simulink model "AircraftModel_LonMot"  (R2020b)
settings: Solver=VariableStepAuto  StartTime=0.0  StopTime=2000  FixedStep=CNT_StepSize  RelTol=1e-3
values from neighbouring files (symbols this model uses):
  CNT_g = 9.81    [AircraftParameters_LonMot.m]
  CNT_m = 15917    [AircraftParameters_LonMot.m]
undefined symbols (not defined in the file or in its folder): Actuators, ControlLaws, Propulsion, TrimPoint
libraries: simulink x19, vrlib x2
settings Model: Creator=NicolasS  LastModifiedBy=vlsag
settings DataIOCC: ExternalInput=getinputstruct(spec1)  InitialState=getstatestruct(spec1)
settings DebuggingCC: BusObjectLabelMismatch=none

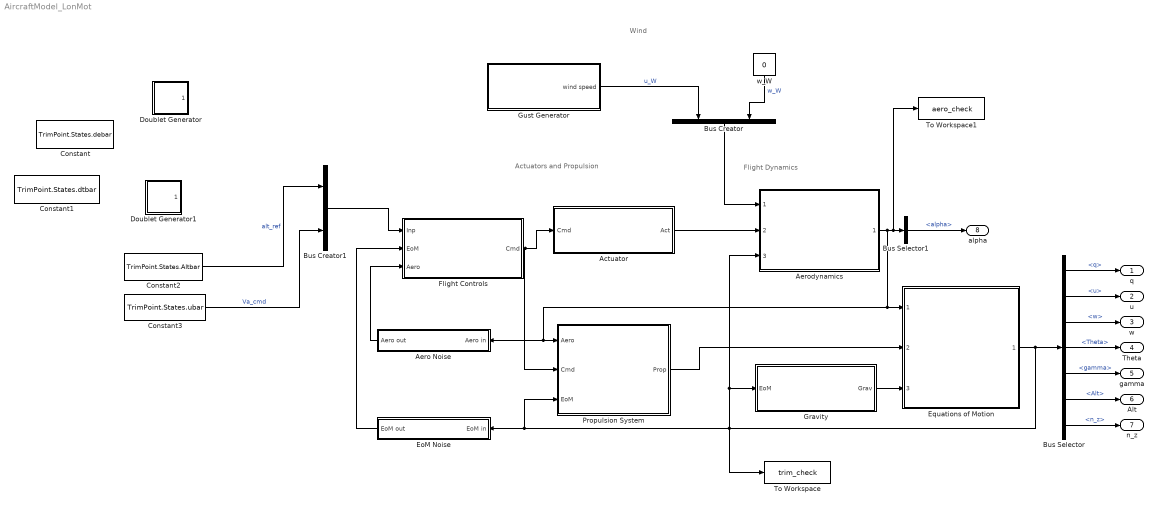
== system AircraftModel_LonMot ==
  note: Wind
  note: Actuators and Propulsion
  note: Flight Dynamics
  Actuator : Subsystem
  Aero Noise : Subsystem
  Aerodynamics : Subsystem  ReferencedSubsystem=Aerodyn
  Bus Creator : BusCreator  Inputs=2  OutDataTypeStr=Bus: WaT
  Bus Creator1 : BusCreator  Inputs=2
  Bus Selector : BusSelector  OutputSignals=q,vv_f.u,vv_f.w,Theta,gamma,Alt,nn_f.n_z
  Bus Selector1 : BusSelector  OutputSignals=AirData.alpha
  Constant : Constant  Value=TrimPoint.States.debar  VectorParams1D=off  SampleTime=-1
  Constant1 : Constant  Value=TrimPoint.States.dtbar  SampleTime=-1
  Constant2 : Constant  Value=TrimPoint.States.Altbar
  Constant3 : Constant  Value=TrimPoint.States.ubar
  Doublet Generator : Subsystem  mask(DoubletGenerator){timeon=25, pulsewidth=20, amplitude=5}
      mask prompts: timeon "Time Start"; pulsewidth "Pulse Duration"
      mask help:
      | Doublet Generator.
      | Ouputs doublet of specificed amplitude and duration.
      |
      | If start/duration/amplitude parameters are vectors, then output is multichannel.
      mask Display: plot([.1 .3 .3001 .4 .4001 .5  .5001 .7],[0 0 1 1 -1 -1 0 0])
  Doublet Generator1 : Subsystem  mask(DoubletGenerator){timeon=10, pulsewidth=40, amplitude=100}
      mask prompts: timeon "Time Start"; pulsewidth "Pulse Duration"
      mask help:
      | Doublet Generator.
      | Ouputs doublet of specificed amplitude and duration.
      |
      | If start/duration/amplitude parameters are vectors, then output is multichannel.
      mask Display: plot([.1 .3 .3001 .4 .4001 .5  .5001 .7],[0 0 1 1 -1 -1 0 0])
  EoM Noise : Subsystem
  Equations of Motion : Subsystem  ReferencedSubsystem=Equations_of_Motion
  Flight Controls : Subsystem
  Gravity : Subsystem
  Gust Generator : Subsystem  mask{gust_start=10, gust_duration=25, gust_amplitude=15}
      mask prompts: gust_start "start time of the gust in sec"; gust_duration "gust duration in sec"; gust_amplitude "maximum gust speed in m/s"
      mask DialogControl ParameterGroupVar Prompt: gust characteristics
  Propulsion System : Subsystem
  To Workspace : ToWorkspace  VariableName=trim_check  SaveFormat=Timeseries  SampleTime=-1
      settings: Decimation=2
  To Workspace1 : ToWorkspace  VariableName=aero_check  SaveFormat=Timeseries  SampleTime=-1
      settings: Decimation=2
  w_W : Constant  Value=0  SampleTime=-1
  q : Outport
  u : Outport  Port=2
  w : Outport  Port=3
  Theta : Outport  Port=4
  gamma : Outport  Port=5
  Alt : Outport  Port=6
  n_z : Outport  Port=7
  alpha : Outport  Port=8
  wires:
  Actuator/1(Act) -> Aerodynamics/2
  w_W/1 -> Bus Creator/2  "w_W"
  Propulsion System/1(Prop) -> Equations of Motion/2
  Bus Selector/6 -> Alt/1  "<Alt>"
  Bus Selector/1 -> q/1  "<q>"
  Bus Selector/2 -> u/1  "<u>"
  Bus Selector/3 -> w/1  "<w>"
  Bus Selector/4 -> Theta/1  "<Theta>"
  Bus Selector/7 -> n_z/1  "<n_z>"
  Bus Selector1/1 -> alpha/1  "<alpha>"
  Gravity/1(Grav) -> Equations of Motion/3
  Bus Selector/5 -> gamma/1  "<gamma>"
  Bus Creator/1 -> Aerodynamics/1
  Flight Controls/1(Cmd) -> Propulsion System/2(Cmd), Actuator/1(Cmd)
  Aerodynamics/1 -> To Workspace1/1, Bus Selector1/1, Aero Noise/1(Aero in), Propulsion System/1(Aero), Equations of Motion/1
  Equations of Motion/1 -> To Workspace/1, Propulsion System/3(EoM), EoM Noise/1(EoM in), Aerodynamics/3, Gravity/1(EoM), Bus Selector/1
  Gust Generator/1(wind speed) -> Bus Creator/1  "u_W"
  EoM Noise/1(EoM out) -> Flight Controls/2(EoM)
  Aero Noise/1(Aero out) -> Flight Controls/3(Aero)
  Bus Creator1/1 -> Flight Controls/1(Inp)
  Constant3/1 -> Bus Creator1/2  "Va_cmd"
  Constant2/1 -> Bus Creator1/1  "alt_ref"

== system AircraftModel_LonMot/Actuator ==
  Cmd : Inport  OutDataTypeStr=Bus: Cmd
  Bus Creator : BusCreator  Inputs=1  OutDataTypeStr=Bus: Act
  Bus Selector : BusSelector  OutputSignals=cmd_de
  Saturation : Saturate  UpperLimit=0.2332  LowerLimit=-0.3115
  State-Space : StateSpace  A=Actuators.Act_e.A  B=Actuators.Act_e.B  C=Actuators.Act_e.C  D=Actuators.Act_e.D  InitialCondition=TrimPoint.States.debar  ContinuousStateAttributes='de'
  Transport Delay : TransportDelay  DelayTime=0.033  InitialOutput=TrimPoint.States.debar  TransDelayFeedthrough=on
  Act : Outport  OutDataTypeStr=Bus: Act
  wires:
  Bus Creator/1 -> Act/1  "Act"
  Cmd/1 -> Bus Selector/1
  State-Space/1 -> Saturation/1  "de"
  Bus Selector/1 -> Transport Delay/1  "<cmd_de>"
  Saturation/1 -> Bus Creator/1  "de"
  Transport Delay/1 -> State-Space/1

== system AircraftModel_LonMot/Aero Noise ==
  Aero in : Inport  OutDataTypeStr=Bus: Aero
  Band-Limited White Noise8 : simulink/Sources/Band-Limited White Noise  Cov=1E-7  Ts=0.01  seed=3324
  Band-Limited White Noise9 : simulink/Sources/Band-Limited White Noise  Cov=1E-3  Ts=0.05  seed=8153
  Bus Creator2 : BusCreator  Inputs=4  OutDataTypeStr=Bus: Aero
  Bus Creator3 : BusCreator  Inputs=5  OutDataTypeStr=Bus: AirData
  Bus Selector : BusSelector  OutputSignals=AirData.u_Af,AirData.w_Af,AirData.V_A,AirData.p_dyn,AirData.alpha,X_Af,Z_Af,M_Af
  Sum1 : Sum  Inputs=++|
  Sum3 : Sum  Inputs=++|
  Aero out : Outport  OutDataTypeStr=Bus: Aero
  wires:
  Aero in/1 -> Bus Selector/1
  Bus Creator3/1 -> Bus Creator2/1  "AirData"
  Bus Selector/6 -> Bus Creator2/2  "<X_Af>"
  Bus Selector/7 -> Bus Creator2/3  "<Z_Af>"
  Bus Selector/8 -> Bus Creator2/4  "<M_Af>"
  Bus Creator2/1 -> Aero out/1  "Aero"
  Bus Selector/1 -> Bus Creator3/1  "<u_Af>"
  Bus Selector/2 -> Bus Creator3/2  "<w_Af>"
  Bus Selector/3 -> Sum3/2  "<V_A>"
  Bus Selector/5 -> Sum1/2  "<alpha>"
  Band-Limited White Noise8/1 -> Sum1/1
  Sum1/1 -> Bus Creator3/5  "alpha"
  Bus Selector/4 -> Bus Creator3/4  "<p_dyn>"
  Band-Limited White Noise9/1 -> Sum3/1
  Sum3/1 -> Bus Creator3/3  "V_A"

== system AircraftModel_LonMot/Doublet Generator ==
  Add : Sum  Inputs=+++
  DownStep : Step  Time=timeon+pulsewidth  After=-2  SampleTime=0
  Gain : Gain  Gain=amplitude
  UnStep : Step  Time=timeon+2*pulsewidth  SampleTime=0
  UpStep : Step  Time=timeon  SampleTime=0
  Doublet : Outport
  wires:
  UpStep/1 -> Add/1
  DownStep/1 -> Add/2
  UnStep/1 -> Add/3
  Add/1 -> Gain/1
  Gain/1 -> Doublet/1

== system AircraftModel_LonMot/Doublet Generator1 ==
  Add : Sum  Inputs=+++
  DownStep : Step  Time=timeon+pulsewidth  After=-2  SampleTime=0
  Gain : Gain  Gain=amplitude
  UnStep : Step  Time=timeon+2*pulsewidth  SampleTime=0
  UpStep : Step  Time=timeon  SampleTime=0
  Doublet : Outport
  wires:
  UpStep/1 -> Add/1
  DownStep/1 -> Add/2
  UnStep/1 -> Add/3
  Add/1 -> Gain/1
  Gain/1 -> Doublet/1

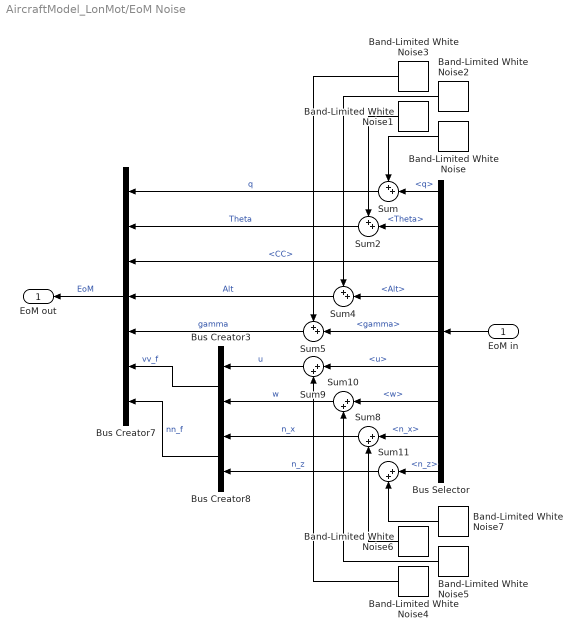
== system AircraftModel_LonMot/EoM Noise ==
  EoM in : Inport  OutDataTypeStr=Bus: EoM
  Band-Limited White Noise : simulink/Sources/Band-Limited White Noise  Cov=1E-5  Ts=0.01  seed=[23341]
  Band-Limited White Noise1 : simulink/Sources/Band-Limited White Noise  Cov=5E-7  Ts=0.01  seed=45875
  Band-Limited White Noise2 : simulink/Sources/Band-Limited White Noise  Cov=1E-4  Ts=0.1  seed=6874
  Band-Limited White Noise3 : simulink/Sources/Band-Limited White Noise  Cov=1E-7  Ts=0.01  seed=8153
  Band-Limited White Noise4 : simulink/Sources/Band-Limited White Noise  Cov=5E-5  Ts=0.1  seed=54769
  Band-Limited White Noise5 : simulink/Sources/Band-Limited White Noise  Cov=1E-4  Ts=0.01  seed=6932
  Band-Limited White Noise6 : simulink/Sources/Band-Limited White Noise  Cov=1E-5  Ts=0.01  seed=11452
  Band-Limited White Noise7 : simulink/Sources/Band-Limited White Noise  Cov=1E-5  Ts=0.01  seed=3324
  Bus Creator3 : BusCreator  Inputs=2  OutDataTypeStr=Bus: vv_f
  Bus Creator7 : BusCreator  Inputs=7  OutDataTypeStr=Bus: EoM
  Bus Creator8 : BusCreator  Inputs=2  OutDataTypeStr=Bus: nn_f
  Bus Selector : BusSelector  OutputSignals=q,Theta,CC,Alt,gamma,vv_f.u,vv_f.w,nn_f.n_x,nn_f.n_z
  Sum{,2,4..5} (4 alike) : Sum  Inputs=++|
  Sum{8..11} (4 alike) : Sum  Inputs=|++
  EoM out : Outport  OutDataTypeStr=Bus: EoM
  wires:
  Bus Selector/3 -> Bus Creator7/3  "<CC>"
  Bus Selector/9 -> Sum11/1  "<n_z>"
  Sum5/1 -> Bus Creator7/5  "gamma"
  Bus Creator8/1 -> Bus Creator7/7  "nn_f"
  Sum8/1 -> Bus Creator8/1  "n_x"
  Band-Limited White Noise/1 -> Sum/1
  Bus Selector/5 -> Sum5/2  "<gamma>"
  EoM in/1 -> Bus Selector/1
  Bus Selector/4 -> Sum4/2  "<Alt>"
  Bus Creator7/1 -> EoM out/1  "EoM"
  Band-Limited White Noise5/1 -> Sum10/2
  Bus Selector/8 -> Sum8/1  "<n_x>"
  Bus Creator3/1 -> Bus Creator7/6  "vv_f"
  Sum2/1 -> Bus Creator7/2  "Theta"
  Sum9/1 -> Bus Creator3/1  "u"
  Sum11/1 -> Bus Creator8/2  "n_z"
  Band-Limited White Noise3/1 -> Sum5/1
  Sum/1 -> Bus Creator7/1  "q"
  Band-Limited White Noise2/1 -> Sum4/1
  Bus Selector/6 -> Sum9/1  "<u>"
  Bus Selector/2 -> Sum2/2  "<Theta>"
  Band-Limited White Noise7/1 -> Sum11/2
  Bus Selector/7 -> Sum10/1  "<w>"
  Band-Limited White Noise4/1 -> Sum9/2
  Band-Limited White Noise1/1 -> Sum2/1
  Band-Limited White Noise6/1 -> Sum8/2
  Sum10/1 -> Bus Creator3/2  "w"
  Bus Selector/1 -> Sum/2  "<q>"
  Sum4/1 -> Bus Creator7/4  "Alt"

== system AircraftModel_LonMot/Flight Controls ==
  Inp : Inport
  EoM : Inport  Port=2  OutDataTypeStr=Bus: EoM
  Aero : Inport  Port=3  OutDataTypeStr=Bus: Aero
  Bus Creator2 : BusCreator  Inputs=2  OutDataTypeStr=Bus: Cmd
  Longitudinal Control Laws : Subsystem
  Cmd : Outport
  wires:
  EoM/1 -> Longitudinal Control Laws/2(EoM)
  Bus Creator2/1 -> Cmd/1  "Cmd"
  Longitudinal Control Laws/2(cmd_dt) -> Bus Creator2/2  "cmd_dt"
  Longitudinal Control Laws/1(cmd_de) -> Bus Creator2/1  "cmd_de"
  Inp/1 -> Longitudinal Control Laws/3(Inp)
  Aero/1 -> Longitudinal Control Laws/1(Aero)

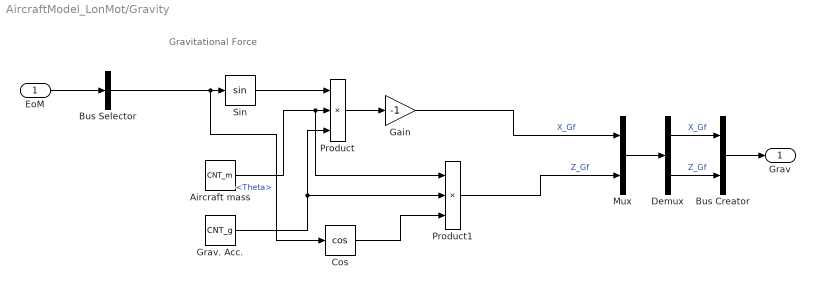
== system AircraftModel_LonMot/Gravity ==
  note: Gravitational Force
  EoM : Inport  OutDataTypeStr=Bus: EoM
  Aircraft mass : Constant  Value=CNT_m  SampleTime=-1
  Bus Creator : BusCreator  Inputs=2  OutDataTypeStr=Bus: Grav
  Bus Selector : BusSelector  OutputSignals=Theta
  Cos : Trigonometry  Operator=cos
  Demux : Demux  Outputs=2
  Gain : Gain  Gain=-1
  Grav. Acc. : Constant  Value=CNT_g  SampleTime=-1
  Mux : Mux  Inputs=2
  Product : Product  Inputs=3
  Product1 : Product  Inputs=3
  Sin : Trigonometry
  Grav : Outport  OutDataTypeStr=Bus: Grav
  wires:
  EoM/1 -> Bus Selector/1
  Demux/1 -> Bus Creator/1  "X_Gf"
  Demux/2 -> Bus Creator/2  "Z_Gf"
  Bus Creator/1 -> Grav/1
  Mux/1 -> Demux/1
  Bus Selector/1 -> Cos/1, Sin/1  "<Theta>"
  Sin/1 -> Product/1
  Aircraft mass/1 -> Product1/1, Product/2
  Grav. Acc./1 -> Product1/2, Product/3
  Product/1 -> Gain/1
  Gain/1 -> Mux/1  "X_Gf"
  Cos/1 -> Product1/3
  Product1/1 -> Mux/2  "Z_Gf"

== system AircraftModel_LonMot/Gust Generator ==
  1-cos gust : Subsystem  TreatAsAtomicUnit=on
  Clock : Clock
  Compare To Constant : simulink/Logic and Bit Operations/Compare To Constant  relop=>=  const=gust_start  OutDataTypeStr=boolean
  Constant : Constant  Value=0
  Sum : Sum  Inputs=+-|
  Switch : Switch  Criteria=u2 > Threshold  Threshold=gust_start+gust_duration
  time freeze : Subsystem  TreatAsAtomicUnit=on
  wind speed : Outport
  wires:
  time freeze/1(out) -> Sum/2
  Constant/1 -> Switch/1
  Clock/1 -> time freeze/1(in), Compare To Constant/1, Sum/1, Switch/2
  Compare To Constant/1 -> 1-cos gust/Enable, time freeze/Trigger
  Sum/1 -> 1-cos gust/1(in)
  1-cos gust/1(wind) -> Switch/3
  Switch/1 -> wind speed/1

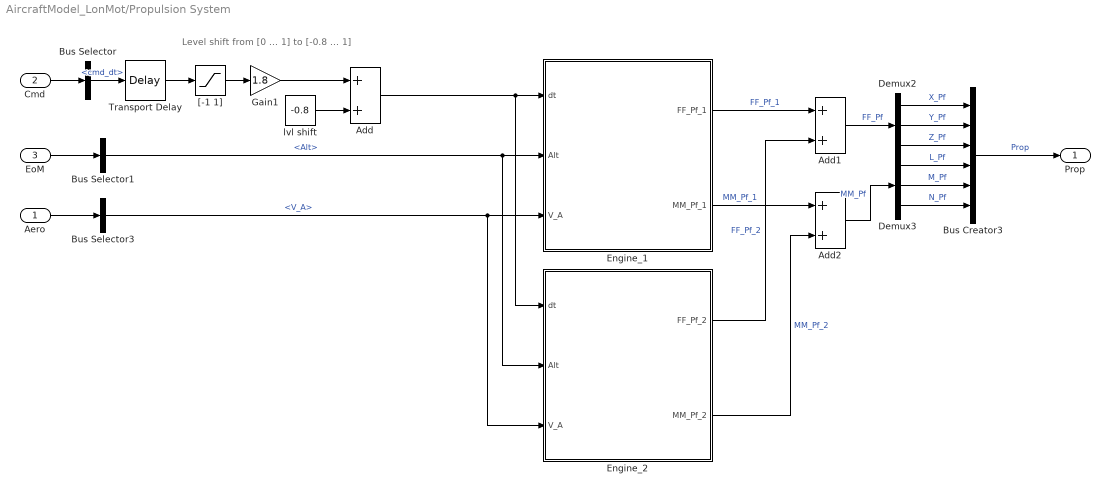
== system AircraftModel_LonMot/Propulsion System ==
  note: Level shift from [0 ... 1] to [-0.8 ... 1]
  Aero : Inport  OutDataTypeStr=Bus: Aero
  Cmd : Inport  Port=2  OutDataTypeStr=Bus: Cmd
  EoM : Inport  Port=3  OutDataTypeStr=Bus: EoM
  Add : Sum
  Add1 : Sum
  Add2 : Sum
  Bus Creator3 : BusCreator  Inputs=6  OutDataTypeStr=Bus: Prop
  Bus Selector : BusSelector  OutputSignals=cmd_dt
  Bus Selector1 : BusSelector  OutputSignals=Alt
  Bus Selector3 : BusSelector  OutputSignals=AirData.V_A
  Demux2 : Demux  Outputs=3
  Demux3 : Demux  Outputs=3
  Engine_1 : Subsystem
  Engine_2 : Subsystem
  Gain1 : Gain  Gain=1.8
  Transport Delay : TransportDelay  DelayTime=0.45  InitialOutput=TrimPoint.States.dtbar  TransDelayFeedthrough=on
  "[-1 1]" : Saturate  UpperLimit=1  LowerLimit=0
  lvl shift : Constant  Value=-0.8  SampleTime=-1
  Prop : Outport  OutDataTypeStr=Bus: Prop
  wires:
  Demux2/2 -> Bus Creator3/2  "Y_Pf"
  Engine_1/1(FF_Pf_1) -> Add1/1  "FF_Pf_1"
  Demux3/1 -> Bus Creator3/4  "L_Pf"
  EoM/1 -> Bus Selector1/1
  lvl shift/1 -> Add/2
  Engine_2/1(FF_Pf_2) -> Add1/2  "FF_Pf_2"
  Add2/1 -> Demux3/1  "MM_Pf"
  Bus Selector3/1 -> Engine_2/3(V_A), Engine_1/3(V_A)  "<V_A>"
  Aero/1 -> Bus Selector3/1
  Demux2/1 -> Bus Creator3/1  "X_Pf"
  Gain1/1 -> Add/1
  Engine_1/2(MM_Pf_1) -> Add2/1  "MM_Pf_1"
  Add/1 -> Engine_2/1(dt), Engine_1/1(dt)
  Bus Creator3/1 -> Prop/1  "Prop"
  Demux3/2 -> Bus Creator3/5  "M_Pf"
  "[-1 1]"/1 -> Gain1/1
  Demux2/3 -> Bus Creator3/3  "Z_Pf"
  Add1/1 -> Demux2/1  "FF_Pf"
  Bus Selector1/1 -> Engine_2/2(Alt), Engine_1/2(Alt)  "<Alt>"
  Demux3/3 -> Bus Creator3/6  "N_Pf"
  Cmd/1 -> Bus Selector/1
  Bus Selector/1 -> Transport Delay/1  "<cmd_dt>"
  Engine_2/2(MM_Pf_2) -> Add2/2  "MM_Pf_2"
  Transport Delay/1 -> "[-1 1]"/1

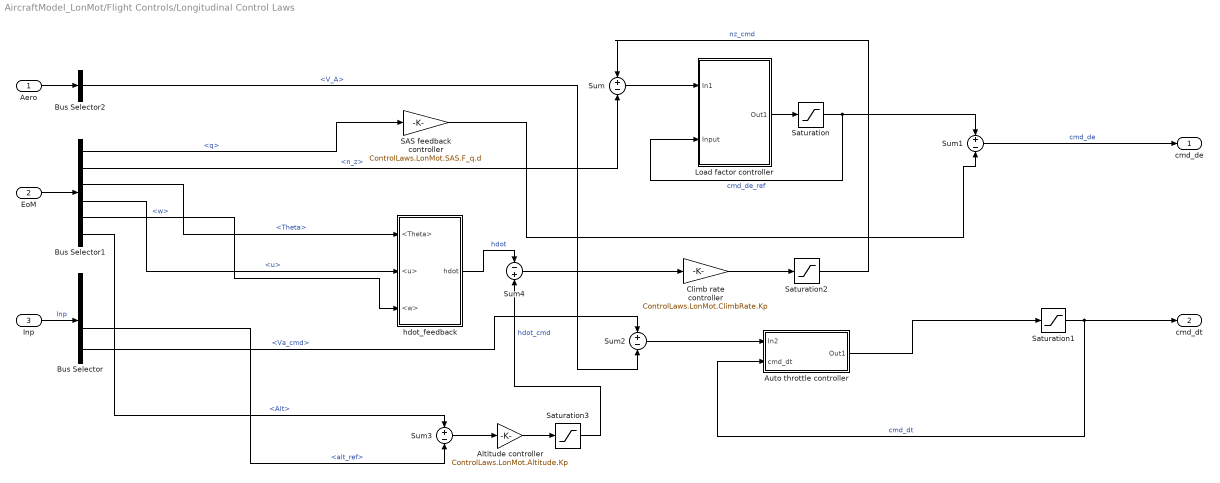
== system AircraftModel_LonMot/Flight Controls/Longitudinal Control Laws ==
  Aero : Inport  OutDataTypeStr=Bus: Aero
  EoM : Inport  Port=2  OutDataTypeStr=Bus: EoM
  Inp : Inport  Port=3
  Altitude controller : Gain  Gain=ControlLaws.LonMot.Altitude.Kp
  Auto throttle controller : Subsystem
  Bus Selector : BusSelector  OutputSignals=hdot_doublet,alt_doublet,alt_ref,Va_cmd
  Bus Selector1 : BusSelector  OutputSignals=q,nn_f.n_z,Theta,vv_f.u,vv_f.w,Alt
  Bus Selector2 : BusSelector  OutputSignals=AirData.V_A
  Climb rate controller : Gain  Gain=ControlLaws.LonMot.ClimbRate.Kp
  Load factor controller : Subsystem
  SAS feedback controller : Gain  Gain=ControlLaws.LonMot.SAS.F_q.d
  Saturation : Saturate  UpperLimit=Actuators.Limits.u_max_He(2)  LowerLimit=Actuators.Limits.u_max_He(1)
  Saturation1 : Saturate  UpperLimit=1  LowerLimit=0
  Saturation2 : Saturate  UpperLimit=ControlLaws.Saturations.nz(2)  LowerLimit=ControlLaws.Saturations.nz(1)  LinearizeAsGain=off
  Saturation3 : Saturate  UpperLimit=ControlLaws.Saturations.hdot(2)  LowerLimit=ControlLaws.Saturations.hdot(1)
  Sum{,1..3} (4 alike) : Sum  Inputs=+-
  Sum4 : Sum  Inputs=-+
  hdot_feedback : Subsystem
  cmd_de : Outport
  cmd_dt : Outport  Port=2
  wires:
  Inp/1 -> Bus Selector/1  "Inp"
  EoM/1 -> Bus Selector1/1
  Bus Selector1/1 -> SAS feedback controller/1  "<q>"
  Aero/1 -> Bus Selector2/1
  Bus Selector1/2 -> Sum/2  "<n_z>"
  Sum/1 -> Load factor controller/1(In1)
  Load factor controller/1(Out1) -> Saturation/1
  Saturation/1 -> Sum1/1, Load factor controller/2(Input)  "cmd_de_ref"
  SAS feedback controller/1 -> Sum1/2
  Sum1/1 -> cmd_de/1  "cmd_de"
  Saturation1/1 -> cmd_dt/1, Auto throttle controller/2(cmd_dt)  "cmd_dt"
  Bus Selector2/1 -> Sum2/2  "<V_A>"
  Sum2/1 -> Auto throttle controller/1(In2)
  Auto throttle controller/1(Out1) -> Saturation1/1
  Bus Selector1/3 -> hdot_feedback/1(<Theta>)  "<Theta>"
  Bus Selector1/4 -> hdot_feedback/2(<u>)  "<u>"
  Bus Selector1/5 -> hdot_feedback/3(<w>)  "<w>"
  Climb rate controller/1 -> Saturation2/1
  Bus Selector1/6 -> Sum3/1  "<Alt>"
  Sum3/1 -> Altitude controller/1
  Altitude controller/1 -> Saturation3/1
  hdot_feedback/1(hdot) -> Sum4/1  "hdot"
  Bus Selector/4 -> Sum2/1  "<Va_cmd>"
  Sum4/1 -> Climb rate controller/1
  Saturation2/1 -> Sum/1  "nz_cmd"
  Bus Selector/3 -> Sum3/2  "<alt_ref>"
  Saturation3/1 -> Sum4/2  "hdot_cmd"

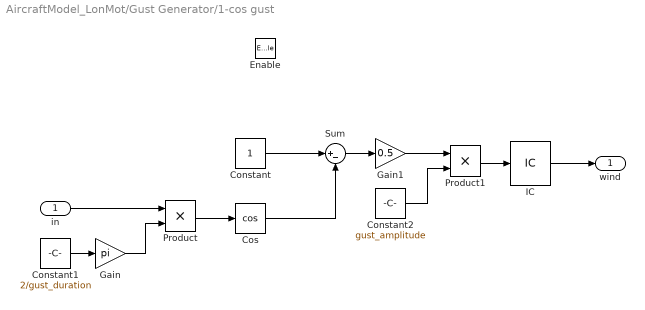
== system AircraftModel_LonMot/Gust Generator/1-cos gust ==
  in : Inport
  Enable : EnablePort  StatesWhenEnabling=reset
  Constant : Constant
  Constant1 : Constant  Value=2/gust_duration
  Constant2 : Constant  Value=gust_amplitude
  Cos : Trigonometry  Operator=cos
  Gain : Gain  Gain=pi
  Gain1 : Gain  Gain=0.5
  IC : InitialCondition  Value=0
  Product : Product
  Product1 : Product
  Sum : Sum  Inputs=|+-
  wind : Outport
  wires:
  IC/1 -> wind/1
  Constant1/1 -> Gain/1
  Product1/1 -> IC/1
  Product/1 -> Cos/1
  Cos/1 -> Sum/2
  Constant/1 -> Sum/1
  Gain/1 -> Product/2
  Gain1/1 -> Product1/1
  Sum/1 -> Gain1/1
  Constant2/1 -> Product1/2
  in/1 -> Product/1

== system AircraftModel_LonMot/Gust Generator/time freeze ==
  in : Inport
  Trigger : TriggerPort  VariantControl=Variant
  out : Outport  InitialOutput=0
  wires:
  in/1 -> out/1

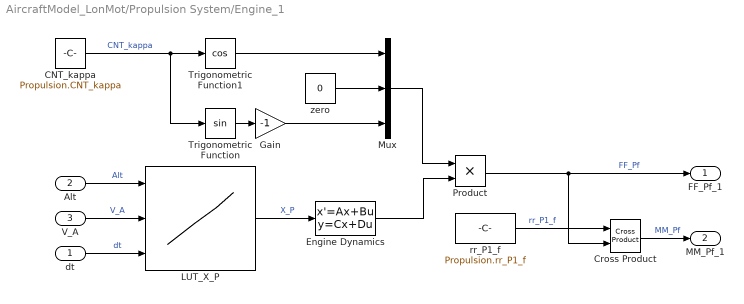
== system AircraftModel_LonMot/Propulsion System/Engine_1 ==
  dt : Inport
  Alt : Inport  Port=2
  V_A : Inport  Port=3
  CNT_kappa : Constant  Value=Propulsion.CNT_kappa  SampleTime=-1
  Cross Product : vrlib/Utilities/Cross Product
  Engine Dynamics : StateSpace  A=Propulsion.Act_t.A  B=Propulsion.Act_t.B  C=Propulsion.Act_t.C  D=Propulsion.Act_t.D  InitialCondition=TrimPoint.States.X_P  ContinuousStateAttributes='X_P1'
  Gain : Gain  Gain=-1
  LUT_X_P : Lookup_n-D  NumberOfTableDimensions=3  BreakpointsForDimension1=Propulsion.LUT.LUT_Alt  BreakpointsForDimension2=Propulsion.LUT.LUT_V_A  BreakpointsForDimension3=Propulsion.LUT.LUT_dt  Table=Propulsion.LUT.LUT_X_P  ExtrapMethod=Clip  InputSameDT=on
      settings: InputPortMap=u0,u1,u2
  Mux : Mux  Inputs=3
  Product : Product  RndMeth=Zero
  Trigonometric Function : Trigonometry
  Trigonometric Function1 : Trigonometry  Operator=cos
  "rr_P1_f " : Constant  Value=Propulsion.rr_P1_f  SampleTime=-1
  zero : Constant  Value=0  SampleTime=-1
  FF_Pf_1 : Outport
  MM_Pf_1 : Outport  Port=2
  wires:
  Alt/1 -> LUT_X_P/1  "Alt"
  V_A/1 -> LUT_X_P/2  "V_A"
  dt/1 -> LUT_X_P/3  "dt"
  zero/1 -> Mux/2
  Mux/1 -> Product/1
  CNT_kappa/1 -> Trigonometric Function1/1, Trigonometric Function/1  "CNT_kappa"
  Trigonometric Function1/1 -> Mux/1
  Product/1 -> FF_Pf_1/1, Cross Product/2  "FF_Pf"
  Cross Product/1 -> MM_Pf_1/1  "MM_Pf"
  Trigonometric Function/1 -> Gain/1
  Gain/1 -> Mux/3
  LUT_X_P/1 -> Engine Dynamics/1  "X_P"
  "rr_P1_f "/1 -> Cross Product/1  "rr_P1_f"
  Engine Dynamics/1 -> Product/2

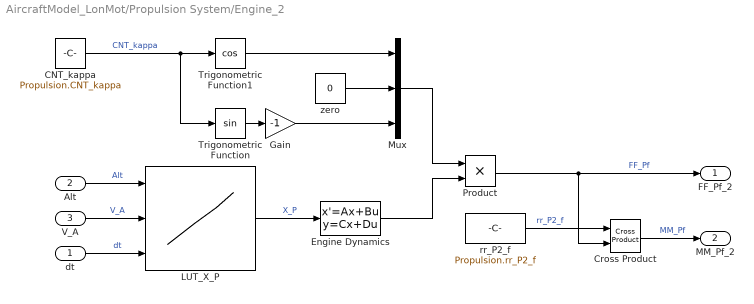
== system AircraftModel_LonMot/Propulsion System/Engine_2 ==
  dt : Inport
  Alt : Inport  Port=2
  V_A : Inport  Port=3
  CNT_kappa : Constant  Value=Propulsion.CNT_kappa  SampleTime=-1
  Cross Product : vrlib/Utilities/Cross Product
  Engine Dynamics : StateSpace  A=Propulsion.Act_t.A  B=Propulsion.Act_t.B  C=Propulsion.Act_t.C  D=Propulsion.Act_t.D  InitialCondition=TrimPoint.States.X_P  ContinuousStateAttributes='X_P2'
  Gain : Gain  Gain=-1
  LUT_X_P : Lookup_n-D  NumberOfTableDimensions=3  BreakpointsForDimension1=Propulsion.LUT.LUT_Alt  BreakpointsForDimension2=Propulsion.LUT.LUT_V_A  BreakpointsForDimension3=Propulsion.LUT.LUT_dt  Table=Propulsion.LUT.LUT_X_P  InputSameDT=on
      settings: InputPortMap=u0,u1,u2
  Mux : Mux  Inputs=3
  Product : Product  RndMeth=Zero
  Trigonometric Function : Trigonometry
  Trigonometric Function1 : Trigonometry  Operator=cos
  "rr_P2_f " : Constant  Value=Propulsion.rr_P2_f  SampleTime=-1
  zero : Constant  Value=0  SampleTime=-1
  FF_Pf_2 : Outport
  MM_Pf_2 : Outport  Port=2
  wires:
  zero/1 -> Mux/2
  Gain/1 -> Mux/3
  Mux/1 -> Product/1
  Cross Product/1 -> MM_Pf_2/1  "MM_Pf"
  Trigonometric Function1/1 -> Mux/1
  Product/1 -> FF_Pf_2/1, Cross Product/2  "FF_Pf"
  Trigonometric Function/1 -> Gain/1
  Alt/1 -> LUT_X_P/1  "Alt"
  dt/1 -> LUT_X_P/3  "dt"
  LUT_X_P/1 -> Engine Dynamics/1  "X_P"
  V_A/1 -> LUT_X_P/2  "V_A"
  "rr_P2_f "/1 -> Cross Product/1  "rr_P2_f"
  CNT_kappa/1 -> Trigonometric Function1/1, Trigonometric Function/1  "CNT_kappa"
  Engine Dynamics/1 -> Product/2

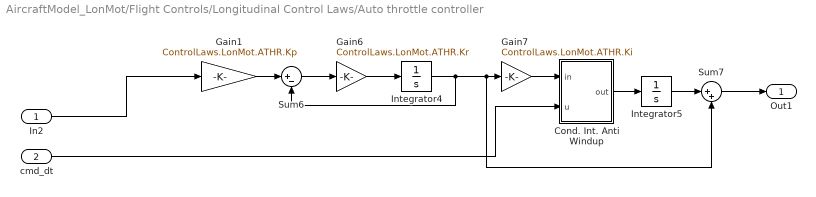
== system AircraftModel_LonMot/Flight Controls/Longitudinal Control Laws/Auto throttle controller ==
  In2 : Inport
  cmd_dt : Inport  Port=2
  Cond. Int. Anti Windup : Subsystem  mask(Integrator Anti-Windup){max_u=inf, min_u=-inf, negative_sign=off}
      mask prompts: max_u "Maximum control signal"; min_u "Minimum control signal"; negative_sign "Negative amplification in control law"
      mask help:
      | This block provides integration using the "conditional integration" anti-windup compensation.
      | It compares the sign of the error and the sign of the control signal and stops integration in case the error drives saturation.
      mask Help:
      | This block provides integration using the "conditional integration" anti-windup compensation. It stops or continues integration depending on the sign of the integrator input (control error) and the commanded control signal. Only if the input would further increase the already saturated integrator output, integration is stopped. This method is different from "integrator clamping" and and "integrator back calculation" and usually provides better recovery properties.
      | 
      | In a standard control architecture the inputs are as follows:
      | INPUT is the error signal r-y
      | RESET is a reset signal. The integrator state is reseted on either rising or falling edges
      | X0 is the initial condition for the integrator
      | U is the commanded control signal
      | 
      | For the anti-windup to work as intended, a saturation block must be placed on the ouput of the control command being fed to the associated actuator, which should include all control signal contributions (e.g. from proportional feedback and inner loops). U is the signal before this saturation.
      | 
      | The default logic assumes a plant with positive steady-state gain to be controlled. This translates to the following logic:
      | For commanded control signal u, saturation limits Umax and Umin, and error e,
      | If u is in bounds, do nothing
      | If u >= Umax AND e > 0, stop integrating
      | If u >= Umax AND e < 0, continue integrating
      | If u <= Umin AND e > 0, continue integrating
      | If u <= Umin AND e < 0, stop integrating
      | 
      | If a plant with negative steady-state gain is to be controlled (e.g. pitch), the windup logic may changed using the NEGATIVE SIGN option. (Note: If unsure check if the controller gains are negative. If yes, check the NEGATIVE SIGN option)
      | This then translates to the logic:
      | If u is in bounds, do nothing
      | If u >= Umax AND e < 0, stop integrating
      | If u >= Umax AND e > 0, continue integrating
      | If u <= Umin AND e < 0, continue integrating
      | If u <= Umin AND e > 0, stop integrating
  Gain1 : Gain  Gain=ControlLaws.LonMot.ATHR.Kp
  Gain6 : Gain  Gain=ControlLaws.LonMot.ATHR.Kr
  Gain7 : Gain  Gain=ControlLaws.LonMot.ATHR.Ki
  Integrator4 : Integrator  UpperSaturationLimit=max(Actuators.Limits.u_max_He)  LowerSaturationLimit=min(Actuators.Limits.u_max_He)  ContinuousStateAttributes='Kathr'
  Integrator5 : Integrator  InitialCondition=TrimPoint.States.dtbar  UpperSaturationLimit=max(Actuators.Limits.u_max_He)  LowerSaturationLimit=min(Actuators.Limits.u_max_He)  ContinuousStateAttributes='Kathr'
  Sum6 : Sum  Inputs=|+-
  Sum7 : Sum  Inputs=|++
  Out1 : Outport
  wires:
  In2/1 -> Gain1/1
  Integrator4/1 -> Sum7/2, Gain7/1, Sum6/2
  cmd_dt/1 -> Cond. Int. Anti Windup/2(u)
  Cond. Int. Anti Windup/1(out) -> Integrator5/1
  Sum6/1 -> Gain6/1
  Gain1/1 -> Sum6/1
  Gain6/1 -> Integrator4/1
  Integrator5/1 -> Sum7/1
  Gain7/1 -> Cond. Int. Anti Windup/1(in)
  Sum7/1 -> Out1/1

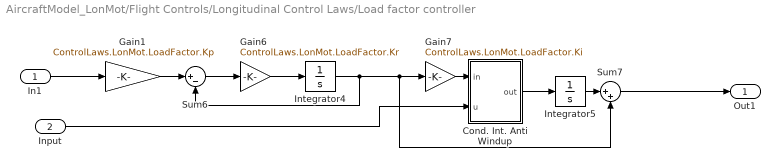
== system AircraftModel_LonMot/Flight Controls/Longitudinal Control Laws/Load factor controller ==
  In1 : Inport
  Input : Inport  Port=2
  Cond. Int. Anti Windup : Subsystem  mask(Integrator Anti-Windup){max_u=inf, min_u=-inf, negative_sign=off}
      mask prompts: max_u "Maximum control signal"; min_u "Minimum control signal"; negative_sign "Negative amplification in control law"
      mask help:
      | This block provides integration using the "conditional integration" anti-windup compensation.
      | It compares the sign of the error and the sign of the control signal and stops integration in case the error drives saturation.
      mask Help:
      | This block provides integration using the "conditional integration" anti-windup compensation. It stops or continues integration depending on the sign of the integrator input (control error) and the commanded control signal. Only if the input would further increase the already saturated integrator output, integration is stopped. This method is different from "integrator clamping" and and "integrator back calculation" and usually provides better recovery properties.
      | 
      | In a standard control architecture the inputs are as follows:
      | INPUT is the error signal r-y
      | RESET is a reset signal. The integrator state is reseted on either rising or falling edges
      | X0 is the initial condition for the integrator
      | U is the commanded control signal
      | 
      | For the anti-windup to work as intended, a saturation block must be placed on the ouput of the control command being fed to the associated actuator, which should include all control signal contributions (e.g. from proportional feedback and inner loops). U is the signal before this saturation.
      | 
      | The default logic assumes a plant with positive steady-state gain to be controlled. This translates to the following logic:
      | For commanded control signal u, saturation limits Umax and Umin, and error e,
      | If u is in bounds, do nothing
      | If u >= Umax AND e > 0, stop integrating
      | If u >= Umax AND e < 0, continue integrating
      | If u <= Umin AND e > 0, continue integrating
      | If u <= Umin AND e < 0, stop integrating
      | 
      | If a plant with negative steady-state gain is to be controlled (e.g. pitch), the windup logic may changed using the NEGATIVE SIGN option. (Note: If unsure check if the controller gains are negative. If yes, check the NEGATIVE SIGN option)
      | This then translates to the logic:
      | If u is in bounds, do nothing
      | If u >= Umax AND e < 0, stop integrating
      | If u >= Umax AND e > 0, continue integrating
      | If u <= Umin AND e < 0, continue integrating
      | If u <= Umin AND e > 0, stop integrating
  Gain1 : Gain  Gain=ControlLaws.LonMot.LoadFactor.Kp
  Gain6 : Gain  Gain=ControlLaws.LonMot.LoadFactor.Kr
  Gain7 : Gain  Gain=ControlLaws.LonMot.LoadFactor.Ki
  Integrator4 : Integrator  UpperSaturationLimit=max(Actuators.Limits.u_max_He)  LowerSaturationLimit=min(Actuators.Limits.u_max_He)  ContinuousStateAttributes='Knz'
  Integrator5 : Integrator  InitialCondition=TrimPoint.States.debar  UpperSaturationLimit=max(Actuators.Limits.u_max_He)  LowerSaturationLimit=min(Actuators.Limits.u_max_He)  ContinuousStateAttributes='Knz'
  Sum6 : Sum  Inputs=|+-
  Sum7 : Sum  Inputs=|++
  Out1 : Outport
  wires:
  Sum6/1 -> Gain6/1
  In1/1 -> Gain1/1
  Gain6/1 -> Integrator4/1
  Gain1/1 -> Sum6/1
  Integrator4/1 -> Gain7/1, Sum7/2, Sum6/2
  Gain7/1 -> Cond. Int. Anti Windup/1(in)
  Integrator5/1 -> Sum7/1
  Sum7/1 -> Out1/1
  Cond. Int. Anti Windup/1(out) -> Integrator5/1
  Input/1 -> Cond. Int. Anti Windup/2(u)

== system AircraftModel_LonMot/Flight Controls/Longitudinal Control Laws/hdot_feedback ==
  <Theta> : Inport
  <u> : Inport  Port=2
  <w> : Inport  Port=3
  Cos : Trigonometry  Operator=cos
  Product : Product
  Product1 : Product
  Sin : Trigonometry
  Sum3 : Sum  Inputs=+-
  hdot : Outport
  wires:
  Product/1 -> Sum3/1
  Cos/1 -> Product1/1
  <Theta>/1 -> Sin/1, Cos/1
  Product1/1 -> Sum3/2
  <w>/1 -> Product1/2
  Sin/1 -> Product/1
  Sum3/1 -> hdot/1
  <u>/1 -> Product/2

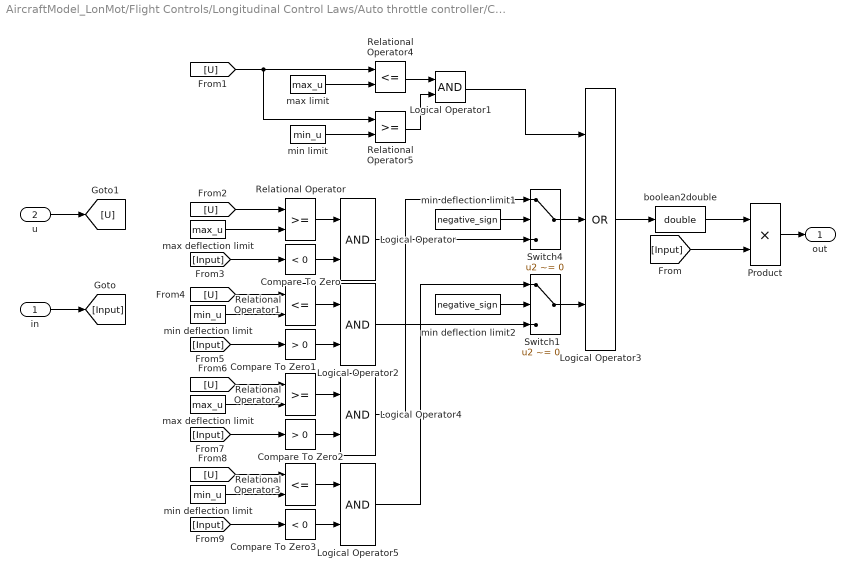
== system AircraftModel_LonMot/Flight Controls/Longitudinal Control Laws/Auto throttle controller/Cond. Int. Anti Windup ==
  in : Inport
  u : Inport  Port=2
  Compare To Zero : simulink/Logic and Bit Operations/Compare To Zero  relop=<  OutDataTypeStr=uint8
  Compare To Zero1 : simulink/Logic and Bit Operations/Compare To Zero  relop=>  OutDataTypeStr=uint8
  Compare To Zero2 : simulink/Logic and Bit Operations/Compare To Zero  relop=>  OutDataTypeStr=uint8
  Compare To Zero3 : simulink/Logic and Bit Operations/Compare To Zero  relop=<  OutDataTypeStr=uint8
  Logical Operator{,1..2,4..5} (5 alike) : Logic  AllPortsSameDT=off  OutDataTypeStr=boolean
  Logical Operator3 : Logic  Operator=OR  Inputs=3  AllPortsSameDT=off  OutDataTypeStr=boolean
  Product : Product
  Relational Operator : RelationalOperator  OutDataTypeStr=boolean  RndMeth=Nearest
  Relational Operator1 : RelationalOperator  Operator=<=  OutDataTypeStr=boolean  RndMeth=Nearest
  Relational Operator2 : RelationalOperator  OutDataTypeStr=boolean  RndMeth=Nearest
  Relational Operator3 : RelationalOperator  Operator=<=  OutDataTypeStr=boolean  RndMeth=Nearest
  Relational Operator4 : RelationalOperator  Operator=<=  OutDataTypeStr=boolean  RndMeth=Nearest
  Relational Operator5 : RelationalOperator  OutDataTypeStr=boolean  RndMeth=Nearest
  Switch1 : Switch  Criteria=u2 ~= 0
  Switch4 : Switch  Criteria=u2 ~= 0
  boolean2double : DataTypeConversion  OutDataTypeStr=double
  max deflection limit : Constant  Value=max_u  SampleTime=-1
  "max deflection limit " : Constant  Value=max_u  SampleTime=-1
  max limit : Constant  Value=max_u  SampleTime=-1
  min deflection limit : Constant  Value=min_u  SampleTime=-1
  "min deflection limit " : Constant  Value=min_u  SampleTime=-1
  min deflection limit1 : Constant  Value=negative_sign  SampleTime=-1
  min deflection limit2 : Constant  Value=negative_sign  SampleTime=-1
  min limit : Constant  Value=min_u  SampleTime=-1
  out : Outport
  wires:
  Product/1 -> out/1
  Logical Operator3/1 -> boolean2double/1
  boolean2double/1 -> Product/1
  [Input] -> Product/2
  [Input] -> Compare To Zero3/1
  [U] -> Relational Operator3/1
  [Input] -> Compare To Zero2/1
  [U] -> Relational Operator2/1
  [Input] -> Compare To Zero1/1
  [U] -> Relational Operator1/1
  [Input] -> Compare To Zero/1
  [U] -> Relational Operator/1
  [U] -> Relational Operator4/1, Relational Operator5/1
  u/1 -> [U]
  in/1 -> [Input]
  min limit/1 -> Relational Operator5/2
  Relational Operator5/1 -> Logical Operator1/2
  Relational Operator4/1 -> Logical Operator1/1
  max limit/1 -> Relational Operator4/2
  Logical Operator5/1 -> Switch1/1
  Logical Operator4/1 -> Switch4/1
  Logical Operator2/1 -> Switch1/3
  Logical Operator/1 -> Switch4/3
  min deflection limit1/1 -> Switch4/2
  Switch1/1 -> Logical Operator3/3
  min deflection limit2/1 -> Switch1/2
  max deflection limit/1 -> Relational Operator/2
  Compare To Zero/1 -> Logical Operator/2
  Relational Operator/1 -> Logical Operator/1
  Compare To Zero1/1 -> Logical Operator2/2
  Relational Operator1/1 -> Logical Operator2/1
  min deflection limit/1 -> Relational Operator1/2
  Switch4/1 -> Logical Operator3/2
  Logical Operator1/1 -> Logical Operator3/1
  Compare To Zero2/1 -> Logical Operator4/2
  Relational Operator2/1 -> Logical Operator4/1
  Compare To Zero3/1 -> Logical Operator5/2
  Relational Operator3/1 -> Logical Operator5/1
  "min deflection limit "/1 -> Relational Operator3/2
  "max deflection limit "/1 -> Relational Operator2/2

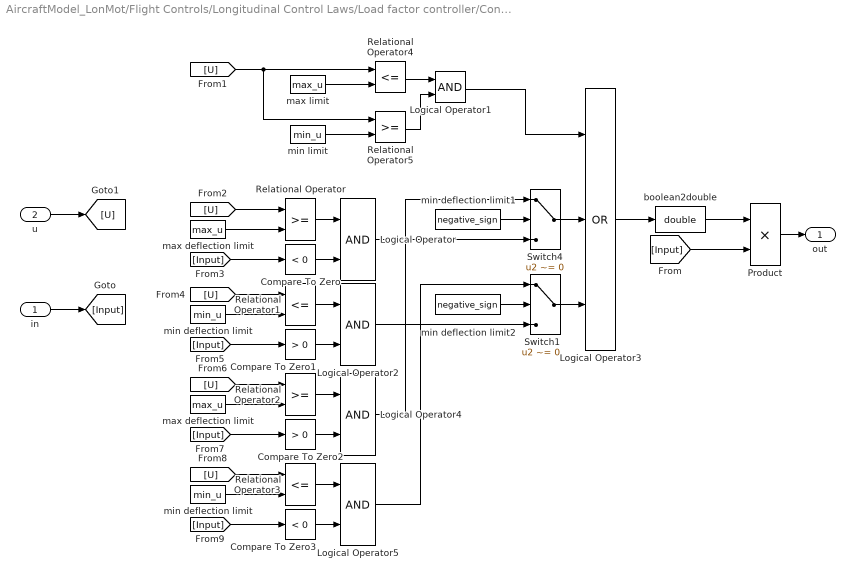
== system AircraftModel_LonMot/Flight Controls/Longitudinal Control Laws/Load factor controller/Cond. Int. Anti Windup ==
  in : Inport
  u : Inport  Port=2
  Compare To Zero : simulink/Logic and Bit Operations/Compare To Zero  relop=<  OutDataTypeStr=uint8
  Compare To Zero1 : simulink/Logic and Bit Operations/Compare To Zero  relop=>  OutDataTypeStr=uint8
  Compare To Zero2 : simulink/Logic and Bit Operations/Compare To Zero  relop=>  OutDataTypeStr=uint8
  Compare To Zero3 : simulink/Logic and Bit Operations/Compare To Zero  relop=<  OutDataTypeStr=uint8
  Logical Operator{,1..2,4..5} (5 alike) : Logic  AllPortsSameDT=off  OutDataTypeStr=boolean
  Logical Operator3 : Logic  Operator=OR  Inputs=3  AllPortsSameDT=off  OutDataTypeStr=boolean
  Product : Product
  Relational Operator : RelationalOperator  OutDataTypeStr=boolean  RndMeth=Nearest
  Relational Operator1 : RelationalOperator  Operator=<=  OutDataTypeStr=boolean  RndMeth=Nearest
  Relational Operator2 : RelationalOperator  OutDataTypeStr=boolean  RndMeth=Nearest
  Relational Operator3 : RelationalOperator  Operator=<=  OutDataTypeStr=boolean  RndMeth=Nearest
  Relational Operator4 : RelationalOperator  Operator=<=  OutDataTypeStr=boolean  RndMeth=Nearest
  Relational Operator5 : RelationalOperator  OutDataTypeStr=boolean  RndMeth=Nearest
  Switch1 : Switch  Criteria=u2 ~= 0
  Switch4 : Switch  Criteria=u2 ~= 0
  boolean2double : DataTypeConversion  OutDataTypeStr=double
  max deflection limit : Constant  Value=max_u  SampleTime=-1
  "max deflection limit " : Constant  Value=max_u  SampleTime=-1
  max limit : Constant  Value=max_u  SampleTime=-1
  min deflection limit : Constant  Value=min_u  SampleTime=-1
  "min deflection limit " : Constant  Value=min_u  SampleTime=-1
  min deflection limit1 : Constant  Value=negative_sign  SampleTime=-1
  min deflection limit2 : Constant  Value=negative_sign  SampleTime=-1
  min limit : Constant  Value=min_u  SampleTime=-1
  out : Outport
  wires:
  Product/1 -> out/1
  Logical Operator3/1 -> boolean2double/1
  boolean2double/1 -> Product/1
  [Input] -> Product/2
  [Input] -> Compare To Zero3/1
  [U] -> Relational Operator3/1
  [Input] -> Compare To Zero2/1
  [U] -> Relational Operator2/1
  [Input] -> Compare To Zero1/1
  [U] -> Relational Operator1/1
  [Input] -> Compare To Zero/1
  [U] -> Relational Operator/1
  [U] -> Relational Operator4/1, Relational Operator5/1
  u/1 -> [U]
  in/1 -> [Input]
  min limit/1 -> Relational Operator5/2
  Relational Operator5/1 -> Logical Operator1/2
  Relational Operator4/1 -> Logical Operator1/1
  max limit/1 -> Relational Operator4/2
  Logical Operator5/1 -> Switch1/1
  Logical Operator4/1 -> Switch4/1
  Logical Operator2/1 -> Switch1/3
  Logical Operator/1 -> Switch4/3
  min deflection limit1/1 -> Switch4/2
  Switch1/1 -> Logical Operator3/3
  min deflection limit2/1 -> Switch1/2
  max deflection limit/1 -> Relational Operator/2
  Compare To Zero/1 -> Logical Operator/2
  Relational Operator/1 -> Logical Operator/1
  Compare To Zero1/1 -> Logical Operator2/2
  Relational Operator1/1 -> Logical Operator2/1
  min deflection limit/1 -> Relational Operator1/2
  Switch4/1 -> Logical Operator3/2
  Logical Operator1/1 -> Logical Operator3/1
  Compare To Zero2/1 -> Logical Operator4/2
  Relational Operator2/1 -> Logical Operator4/1
  Compare To Zero3/1 -> Logical Operator5/2
  Relational Operator3/1 -> Logical Operator5/1
  "min deflection limit "/1 -> Relational Operator3/2
  "max deflection limit "/1 -> Relational Operator2/2
